simulink model "IDMF_datagenerator"  (R2022a)
settings: Solver=VariableStepAuto  StartTime=0.0  StopTime=30  FixedStep=0.05  RelTol=1e-3
PostLoadFcn:
  | %Add subfolders to path
  | addpath('virtualworld');
InitFcn:
  | startScript;
values from neighbouring files (symbols this model uses):
  angularVelocity = [0 0 -0.01]    [startScript.m]
  angularVelocityforLanding = [0 0 0]    [startScript.m]
  dronestartlocation = [-1.5 0 4]    [startScript.m]
  Dstar = -0.5    [startScript.m]
  finalHoverHeight = 2.5    [startScript.m]
  helipadLocation = [14 0.6 5]    [startScript.m]
  linearVelocity = [5 0.05 1]    [startScript.m]
  linearVelocityforHover = [0.65 0.05 0.3]    [startScript.m]
  windAVelocity = [0 0.1 0.1]    [startScript.m]
  windLVelocity = [0.1 0 0.3]    [startScript.m]
undefined symbols (not defined in the file or in its folder): fspecial, gcbh, Kanade, Lucas, Rec, SDTV, vrmfunc
libraries: visiontextngfix x11, visionconversions x9, visionanalysis x8, vrlib x7, slpidlib x3, sharedtransform x2, simulink x1
(part 2 of 3)

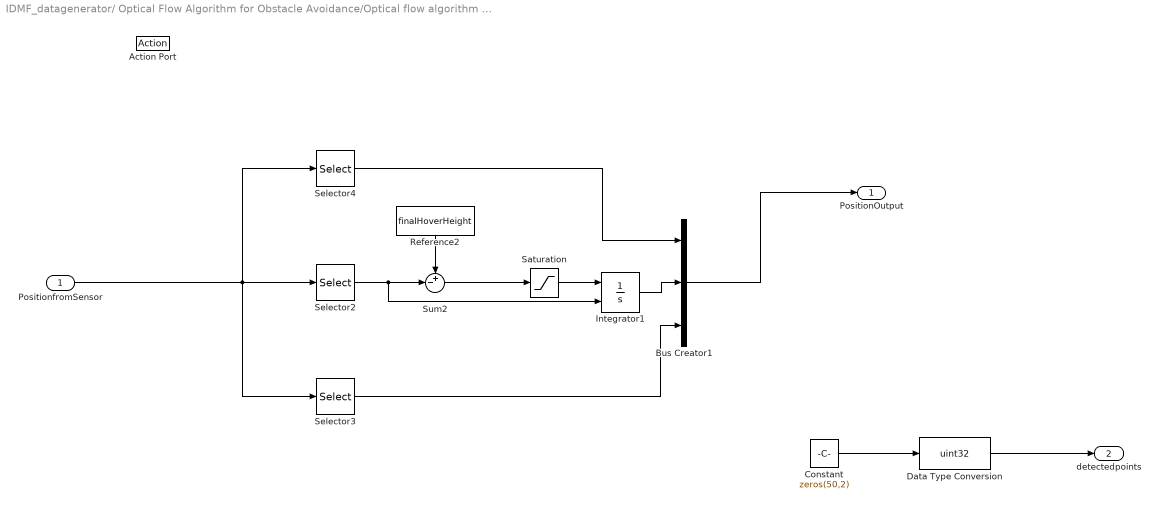
== system IDMF_datagenerator/ Optical Flow Algorithm for Obstacle Avoidance/Optical flow algorithm and PID Controller for landing/DronePositionEstimation.DroneLanding2 ==
  PositionfromSensor : Inport
  Action Port : ActionPort
      settings: CopyFcn=Stateflow.SLINSF.SimulinkMan.removeBlockPreDeleteFcn  PreDeleteFcn=Stateflow.SLINSF.SimulinkMan.unsafePredeleteFcn
  Bus Creator1 : BusCreator  Inputs=3
  Constant : Constant  Value=zeros(50,2)
  Data Type Conversion : DataTypeConversion  OutDataTypeStr=uint32  SaturateOnIntegerOverflow=off  RndMeth=Floor
  Integrator1 : Integrator  InitialConditionSource=external  LimitOutput=on  UpperSaturationLimit=5  LowerSaturationLimit=-5  ZeroCross=off
  Reference2 : Constant  Value=finalHoverHeight
  Saturation : Saturate  UpperLimit=5  LowerLimit=-5
  Selector2 : Selector  InputPortWidth=3  IndexOptions=Index vector (dialog)  Indices=[2]  OutputSizes=1
  Selector3 : Selector  InputPortWidth=3  IndexOptions=Index vector (dialog)  Indices=[3]  OutputSizes=1
  Selector4 : Selector  InputPortWidth=3  IndexOptions=Index vector (dialog)  Indices=[1]  OutputSizes=1
  Sum2 : Sum  Inputs=+-|
  PositionOutput : Outport
  detectedpoints : Outport  Port=2
      settings: VarSizeSig=Yes
  wires:
  Integrator1/1 -> Bus Creator1/2
  Saturation/1 -> Integrator1/1
  Bus Creator1/1 -> PositionOutput/1
  Selector2/1 -> Integrator1/2, Sum2/2
  Selector3/1 -> Bus Creator1/3
  PositionfromSensor/1 -> Selector3/1, Selector4/1, Selector2/1
  Reference2/1 -> Sum2/1
  Selector4/1 -> Bus Creator1/1
  Sum2/1 -> Saturation/1
  Constant/1 -> Data Type Conversion/1
  Data Type Conversion/1 -> detectedpoints/1

== system IDMF_datagenerator/ Optical Flow Algorithm for Obstacle Avoidance/Optical flow algorithm and PID Controller for landing/DronePositionEstimation.DroneLandingnoZ ==
  PositionfromSensor : Inport
  D_est : Inport  Port=2
  camera_d : Inport  Port=3
  linearVelocity : Inport  Port=4
  Action Port : ActionPort
      settings: CopyFcn=Stateflow.SLINSF.SimulinkMan.removeBlockPreDeleteFcn  PreDeleteFcn=Stateflow.SLINSF.SimulinkMan.unsafePredeleteFcn
  Landing : Subsystem
  Subsystem : Subsystem
  PositionOutput : Outport
  detectedpoints : Outport  Port=2  OutDataTypeStr=uint32
  wires:
  PositionfromSensor/1 -> Landing/1(In1)
  D_est/1 -> Landing/2(D_est)
  Landing/1(PositionOutput) -> PositionOutput/1
  camera_d/1 -> Subsystem/1(Input)
  Subsystem/1(Output) -> detectedpoints/1
  linearVelocity/1 -> Landing/3(linearVelocity)

== system IDMF_datagenerator/ Optical Flow Algorithm for Obstacle Avoidance/Optical flow algorithm and PID Controller for landing/DronePositionEstimation.OpticalFlowAlgorithm_ ==
  note: If the output from the Sign block is Positive, drone should move towards the left side, i.e. V_y is Negative. Also, if the output from the Sign block is Negative, drone will move towwars the right side..ie, V_y is Positive.
  note: Steering Linear Velocities
  OpticalFlowDiff : Inport
  Action Port : ActionPort
      settings: CopyFcn=Stateflow.SLINSF.SimulinkMan.removeBlockPreDeleteFcn  PreDeleteFcn=Stateflow.SLINSF.SimulinkMan.unsafePredeleteFcn
  Constant : Constant  Value=uint32(zeros(50,2))
  Constant1 : Constant  Value=linearVelocity
  Gain : Gain  Gain=[1 1 -1]
  Integrator2 : Integrator  InitialCondition=dronestartlocation
  Sign : Signum
  Switch1 : Switch  Criteria=u2 > Threshold  SaturateOnIntegerOverflow=off  InputSameDT=off
  PositionOutput : Outport
  detectedpoints : Outport  Port=2
      settings: VarSizeSig=Yes
  wires:
  OpticalFlowDiff/1 -> Sign/1
  Constant1/1 -> Switch1/3, Gain/1  "[V_X V_Z V_Y]"
  Switch1/1 -> Integrator2/1
  Gain/1 -> Switch1/1  "[V_X V_Z -1*V_Y]"
  Constant/1 -> detectedpoints/1
  Sign/1 -> Switch1/2
  Integrator2/1 -> PositionOutput/1

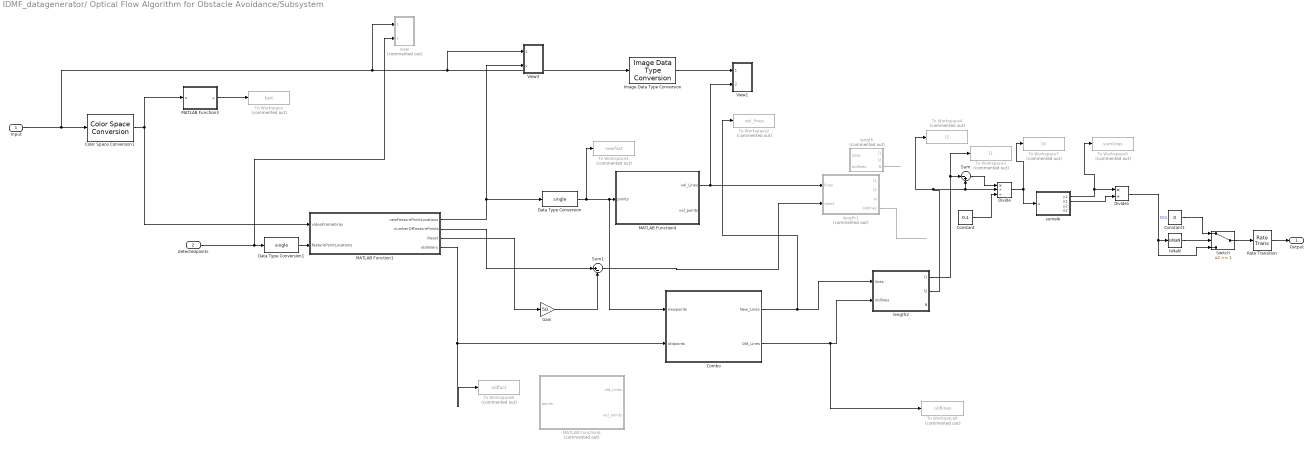
== system IDMF_datagenerator/ Optical Flow Algorithm for Obstacle Avoidance/Subsystem ==
  Input : Inport
  detectedpoints : Inport  Port=2
  Color Space Conversion1 : visionconversions/Color Space  Conversion  conversion=Obsolete  conversionActive=R'G'B' to intensity  wp_str=D65  rec=Rec. 601 (SDTV)  sys=1125/60/2:1  imagePorts=One multidimensional signal
  Combo : MATLAB Function  TreatAsAtomicUnit=on
  Constant : Constant  Value=0.1
  Constant1 : Constant  Value=0
  Data Type Conversion : DataTypeConversion  OutDataTypeStr=single  SaturateOnIntegerOverflow=off  RndMeth=Floor
  Data Type Conversion1 : DataTypeConversion  OutDataTypeStr=single  SaturateOnIntegerOverflow=off  RndMeth=Floor
  Divide : Product  Inputs=*//
  Divide1 : Product  Inputs=*/
  Gain : Gain  Gain=50
  Image Data Type Conversion : visionconversions/Image Data Type Conversion  outDT=single  isSigned=on  wordLen=16  numFracBits=0
      settings: SourceProductBaseCode=VP
  IsNaN : RelationalOperator  Operator=isNaN  OutDataTypeStr=boolean  RndMeth=Simplest  InputSameDT=off
  MATLAB Function1 : MATLAB Function  TreatAsAtomicUnit=on
  MATLAB Function3 : MATLAB Function  TreatAsAtomicUnit=on
  MATLAB Function4 : MATLAB Function  TreatAsAtomicUnit=on
  MATLAB Function6 : MATLAB Function  Commented=on  TreatAsAtomicUnit=on
  Rate Transition : RateTransition  OutPortSampleTime=0.1
  Sum : Sum  Inputs=|-+
  Sum1 : Sum  Inputs=|+-
  Switch : Switch  Threshold=1  SaturateOnIntegerOverflow=off  InputSameDT=off
  To Workspace : ToWorkspace  Commented=on  VariableName=fast  SaveFormat=Timeseries  SampleTime=-1
  To Workspace1 : ToWorkspace  Commented=on  VariableName=newfast  SaveFormat=Timeseries  SampleTime=-1
  To Workspace2 : ToWorkspace  Commented=on  VariableName=vel_lines  SaveFormat=Timeseries  SampleTime=-1
  To Workspace3 : ToWorkspace  Commented=on  VariableName=l1  SaveFormat=Timeseries  SampleTime=-1
  To Workspace4 : ToWorkspace  Commented=on  VariableName=l2  SaveFormat=Timeseries  SampleTime=-1
  To Workspace5 : ToWorkspace  Commented=on  VariableName=sumlines  SaveFormat=Timeseries  SampleTime=-1
  To Workspace6 : ToWorkspace  Commented=on  VariableName=oldlines  SaveFormat=Timeseries  SampleTime=-1
  To Workspace7 : ToWorkspace  Commented=on  VariableName=Di  SaveFormat=Timeseries  SampleTime=-1
  To Workspace8 : ToWorkspace  Commented=on  VariableName=oldfast  SaveFormat=Timeseries  SampleTime=-1
  View : Subsystem  Commented=on
  View1 : Subsystem
  View3 : Subsystem
  length : MATLAB Function  Commented=on  TreatAsAtomicUnit=on
  length1 : MATLAB Function  Commented=on  TreatAsAtomicUnit=on
  length2 : MATLAB Function  TreatAsAtomicUnit=on
  sumele : MATLAB Function  TreatAsAtomicUnit=on
  Output : Outport
  wires:
  Input/1 -> View/1(d_camera), View3/1(d_camera), Image Data Type Conversion/1, Color Space Conversion1/1
  Data Type Conversion/1 -> To Workspace1/1, Combo/1(newpoints), MATLAB Function4/1(points)
  MATLAB Function3/1(y) -> To Workspace/1
  detectedpoints/1 -> View/2(y), Data Type Conversion1/1
  Data Type Conversion1/1 -> MATLAB Function1/2(featurePointLocations)
  Color Space Conversion1/1 -> MATLAB Function1/1(videoFrameGray), MATLAB Function3/1(u)
  Image Data Type Conversion/1 -> View1/1(camera_d)
  Sum/1 -> Divide/1
  Constant/1 -> Divide/3
  Divide/1 -> sumele/1(u), To Workspace7/1
  Divide1/1 -> Switch/3, IsNaN/1  "Dca"
  sumele/1(y1) -> To Workspace5/1, Divide1/1
  sumele/2(n1) -> Divide1/2
  length/3(N) -> ?
  MATLAB Function1/2(numberOfFeaturePoints) -> Sum1/1
  MATLAB Function1/3(Reset) -> Gain/1
  Gain/1 -> Sum1/2
  Sum1/1 -> length1/2(reset)
  MATLAB Function4/1(vel_Lines) -> View1/2(vel_Lines), length1/1(lines)
  length1/4(oldlines) -> ?
  MATLAB Function1/4(oldInliers) -> To Workspace8/1, Combo/2(oldpoints)
  length2/1(l1) -> To Workspace3/1, Sum/1
  length2/2(l2) -> Divide/2, Sum/2, To Workspace4/1
  Combo/2(Old_Lines) -> To Workspace6/1, length2/2(oldlines)
  Combo/1(New_Lines) -> To Workspace2/1, length2/1(lines)
  MATLAB Function1/1(newFeaturePointLocations) -> View3/2(y), Data Type Conversion/1
  IsNaN/1 -> Switch/2
  Switch/1 -> Rate Transition/1
  Constant1/1 -> Switch/1
  Rate Transition/1 -> Output/1

== system IDMF_datagenerator/ Optical Flow Algorithm for Obstacle Avoidance/flowdiff ==
  image : Inport
  Delay1 : Delay
  FlowDifferences : MATLAB Function  TreatAsAtomicUnit=on
  Gain : Gain  Gain=1/10^3
  Sum1 : Sum  Inputs=+-
  Out1 : Outport
  Out2 : Outport  Port=2
  vleftflow : Outport  Port=3
  vrightflow : Outport  Port=4
  cmd : Outport  Port=5
  wires:
  Gain/1 -> Out2/1, Delay1/1, Sum1/1
  FlowDifferences/1(flowDifference) -> Gain/1
  Sum1/1 -> Out1/1
  FlowDifferences/3(vrightflow) -> vrightflow/1
  FlowDifferences/4(cmd) -> cmd/1
  Delay1/1 -> Sum1/2
  image/1 -> FlowDifferences/1(image)
  FlowDifferences/2(vleftflow) -> vleftflow/1

== system IDMF_datagenerator/ Optical Flow Algorithm for Obstacle Avoidance/flowdiff_down ==
  image : Inport
  Delay : Delay  DelayLength=1
  Delay2 : Delay  DelayLength=1
  FlowDifferences1 : MATLAB Function  TreatAsAtomicUnit=on
  FlowDifferences2 : MATLAB Function  TreatAsAtomicUnit=on
  Gain1 : Gain  Gain=1/10^3
  Gain2 : Gain  Gain=1/10^3
  Sum : Sum  Inputs=+-
  Sum2 : Sum  Inputs=+-
  ofd_up_d : Outport
  flowdiff_down : Outport  Port=2
  ofd_d : Outport  Port=3
  flowup_down : Outport  Port=4
  wires:
  image/1 -> FlowDifferences2/1(image), FlowDifferences1/1(image)
  Gain1/1 -> flowdiff_down/1, Sum/1, Delay/1  "flowdiff_down"
  Gain2/1 -> flowup_down/1, Delay2/1, Sum2/1  "flowup_down"
  FlowDifferences1/1(flowDifference) -> Gain1/1  "flowdiff_down"
  Delay/1 -> Sum/2
  FlowDifferences2/1(flowDifference) -> Gain2/1  "flowup_down"
  Sum2/1 -> ofd_up_d/1  "ofd_up_d"
  Delay2/1 -> Sum2/2
  Sum/1 -> ofd_d/1  "ofd_d"

== system IDMF_datagenerator/Optical Flow Lines Calculation/Optical Flow Lines ==
  vel.Values : Inport
  Optical Flow Lines : MATLAB Function  TreatAsAtomicUnit=on
  vel.Lines : Outport
  wires:
  Optical Flow Lines/1(vel_Lines) -> vel.Lines/1
  vel.Values/1 -> Optical Flow Lines/1(vel_Values)

== system IDMF_datagenerator/Optical Flow Lines Calculation/Optical Flow Lines1 ==
  vel.Values : Inport
  Optical Flow Lines : MATLAB Function  TreatAsAtomicUnit=on
  vel.Lines : Outport
  wires:
  Optical Flow Lines/1(vel_Lines) -> vel.Lines/1
  vel.Values/1 -> Optical Flow Lines/1(vel_Values)

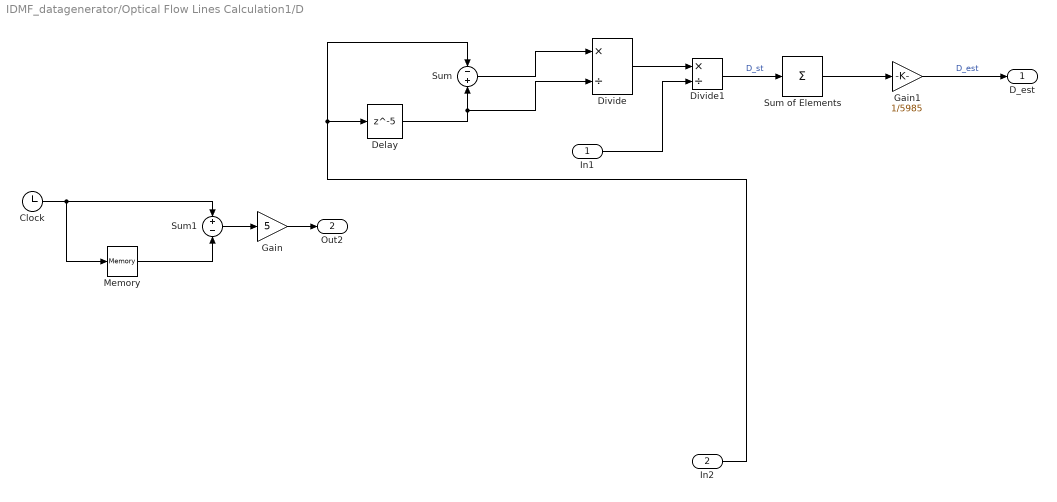
== system IDMF_datagenerator/Optical Flow Lines Calculation1/D ==
  In1 : Inport
  In2 : Inport  Port=2
  Clock : Clock
  Delay : Delay  DelayLength=5
  Divide : Product  Inputs=*/
  Divide1 : Product  Inputs=*/
  Gain : Gain  Gain=5
  Gain1 : Gain  Gain=1/5985
  Memory : Memory
  Sum : Sum  Inputs=-+
  Sum of Elements : Sum  Inputs=+
  Sum1 : Sum  Inputs=+-
  D_est : Outport
  Out2 : Outport  Port=2
  wires:
  Divide/1 -> Divide1/1
  Clock/1 -> Memory/1, Sum1/1
  Sum1/1 -> Gain/1
  Delay/1 -> Divide/2, Sum/2
  Sum/1 -> Divide/1
  Sum of Elements/1 -> Gain1/1
  In2/1 -> Delay/1, Sum/1
  Memory/1 -> Sum1/2
  Divide1/1 -> Sum of Elements/1  "D_st"
  In1/1 -> Divide1/2
  Gain/1 -> Out2/1
  Gain1/1 -> D_est/1  "D_est"

== system IDMF_datagenerator/Optical Flow Lines Calculation1/View ==
  d_camera : Inport
  In2 : Inport  Port=2
  Data Type Conversion : DataTypeConversion  OutDataTypeStr=int32  SaturateOnIntegerOverflow=off  RndMeth=Floor
  Draw Markers1 : visiontextngfix/Draw Markers  shape=X-mark  size=3  fill=off  fillClrSource=Specify via dialog  display=User-specified value  intensity=200  color=[255 0 0]  opacity=0.6  viewport=Entire image  antialiasing=off  inType=Obsolete  imagePorts=One multidimensional signal  roundingMode=Floor  overflowMode=off  memoryMode=Specify word length  memoryWordLength=16  memoryFracLength=15  prodOutputMode=Binary point scaling  prodOutputWordLength=32  prodOutputFracLength=14
      settings: SourceProductBaseCode=VP
  points for ownline : VideoViewer  FigPos=[132 616 560 453]
  wires:
  In2/1 -> Data Type Conversion/1
  Draw Markers1/1 -> points for ownline/1
  d_camera/1 -> Draw Markers1/1
  Data Type Conversion/1 -> Draw Markers1/2

== system IDMF_datagenerator/Optical Flow Lines Calculation1/View1 ==
  In1 : Inport
  In2 : Inport  Port=2
  Data Type Conversion : DataTypeConversion  OutDataTypeStr=int32  SaturateOnIntegerOverflow=off  RndMeth=Floor
  Draw Shapes2 : visiontextngfix/Draw Shapes  shape=Lines  fill=off  lineWidth=1  fillClrSource=Specify via dialog  display=User-specified value  intensity=200  color=[255 255 0]  opacity=0.6  viewport=Entire image  antialiasing=off  inType=Obsolete  imagePorts=One multidimensional signal  roundingMode=Floor  overflowMode=off  memoryMode=Specify word length  memoryWordLength=16  prodOutputMode=Binary point scaling  prodOutputWordLength=32  prodOutputFracLength=14  memoryFracLength=15
  owncode lines : VideoViewer  FigPos=[594 703 418 304]
  wires:
  Draw Shapes2/1 -> owncode lines/1
  In1/1 -> Draw Shapes2/1
  Data Type Conversion/1 -> Draw Shapes2/2
  In2/1 -> Data Type Conversion/1

== system IDMF_datagenerator/ Optical Flow Algorithm for Obstacle Avoidance/Optical flow algorithm and PID Controller for landing/DronePositionEstimation.DroneLandingnoZ/Landing ==
  note: Steering Linear Velocities
  In1 : Inport
  D_est : Inport  Port=2
  linearVelocity : Inport  Port=3
  Bus Creator1 : BusCreator  Inputs=3
  Constant : Constant  Value=linearVelocity
  Integrator2 : Integrator  InitialConditionSource=external  InitialCondition=dronestartlocation
  Manual Switch : ManualSwitch  CurrentSetting=0
  Manual Switch1 : ManualSwitch  CurrentSetting=0
  Selector2 : Selector  InputPortWidth=3  IndexOptions=Index vector (dialog)  Indices=[2]  OutputSizes=1
  Selector3 : Selector  InputPortWidth=3  IndexOptions=Index vector (dialog)  Indices=[3]  OutputSizes=1
  Selector4 : Selector  InputPortWidth=3  IndexOptions=Index vector (dialog)  Indices=[1]  OutputSizes=1
  Subsystem : Subsystem
  PositionOutput : Outport
  wires:
  D_est/1 -> Subsystem/2(D_est)
  Selector4/1 -> Bus Creator1/1
  Selector3/1 -> Bus Creator1/3
  Subsystem/1(Z) -> Bus Creator1/2
  Bus Creator1/1 -> PositionOutput/1
  Selector2/1 -> Subsystem/1(InitialZ)
  Manual Switch/1 -> Integrator2/1  "[V_X V_Z -1*V_Y]"
  Constant/1 -> Manual Switch/1
  Integrator2/1 -> Manual Switch1/1
  linearVelocity/1 -> Manual Switch/2
  Manual Switch1/1 -> Selector4/1, Selector3/1, Selector2/1
  In1/1 -> Integrator2/2, Manual Switch1/2

== system IDMF_datagenerator/ Optical Flow Algorithm for Obstacle Avoidance/Optical flow algorithm and PID Controller for landing/DronePositionEstimation.DroneLandingnoZ/Subsystem ==
  Input : Inport
  Color Space Conversion1 : visionconversions/Color Space  Conversion  conversion=Obsolete  conversionActive=R'G'B' to intensity  wp_str=D65  rec=Rec. 601 (SDTV)  sys=1125/60/2:1  imagePorts=One multidimensional signal
  Corner Detection : visionanalysis/Corner Detection  method=Local intensity comparison (Rosen & Drummond)  factor=0.04  filter=fspecial('gaussian', [1 5], 1.5)  thrInten=0.1  thrAngle=157.5  output=Obsolete9b  outputInUse=Corner location  maxNum=50  thrMetric=0.005  neighborSize=[15 15]  isOutVarDim=off  roundingMode=Floor  overflowMode=off  firstCoeffMode=Specify word length  firstCoeffWordLength=16  firstCoeffFracLength=16  prodOutputMode=Binary point scaling  prodOutputWordLength=32  prodOutputFracLength=0  accumMode=Binary point scaling  accumWordLength=32  accumFracLength=0  memoryMode=Binary point scaling  memoryWordLength=32  memoryFracLength=0
      settings: SourceProductBaseCode=VP
  Corner Detection1 : visionanalysis/Corner Detection  method=Local intensity comparison (Rosen & Drummond)  factor=0.04  filter=fspecial('gaussian', [1 5], 1.5)  thrInten=0.1  thrAngle=112.5  output=Obsolete9b  outputInUse=Corner location  maxNum=50  thrMetric=0.0005  neighborSize=[25 25]  isOutVarDim=off  roundingMode=Floor  overflowMode=off  firstCoeffMode=Specify word length  firstCoeffWordLength=16  firstCoeffFracLength=16  prodOutputMode=Binary point scaling  prodOutputWordLength=32  prodOutputFracLength=0  accumMode=Binary point scaling  accumWordLength=32  accumFracLength=0  memoryMode=Binary point scaling  memoryWordLength=32  memoryFracLength=0
      settings: SourceProductBaseCode=VP
  Output : Outport
  wires:
  Input/1 -> Color Space Conversion1/1
  Color Space Conversion1/1 -> Corner Detection/1
  Corner Detection/1 -> Output/1

== system IDMF_datagenerator/ Optical Flow Algorithm for Obstacle Avoidance/Subsystem/View ==
  d_camera : Inport
  y : Inport  Port=2
  Data Type Conversion : DataTypeConversion  OutDataTypeStr=int32  SaturateOnIntegerOverflow=off  RndMeth=Floor
  Draw Markers1 : visiontextngfix/Draw Markers  shape=X-mark  size=3  fill=off  fillClrSource=Specify via dialog  display=User-specified value  intensity=200  color=[255 0 0]  opacity=0.6  viewport=Entire image  antialiasing=off  inType=Obsolete  imagePorts=One multidimensional signal  roundingMode=Floor  overflowMode=off  memoryMode=Specify word length  memoryWordLength=16  memoryFracLength=15  prodOutputMode=Binary point scaling  prodOutputWordLength=32  prodOutputFracLength=14
      settings: SourceProductBaseCode=VP
  points from new : VideoViewer  FigPos=[1 1038 1920 938]
  wires:
  y/1 -> Data Type Conversion/1
  Draw Markers1/1 -> points from new/1
  d_camera/1 -> Draw Markers1/1
  Data Type Conversion/1 -> Draw Markers1/2

== system IDMF_datagenerator/ Optical Flow Algorithm for Obstacle Avoidance/Subsystem/View1 ==
  camera_d : Inport
  vel_Lines : Inport  Port=2
  Detected lines : VideoViewer  FigPos=[1 1078 1184 528]
  Draw Shapes2 : visiontextngfix/Draw Shapes  shape=Lines  fill=off  lineWidth=1  fillClrSource=Specify via dialog  display=User-specified value  intensity=200  color=[255 255 0]  opacity=0.6  viewport=Entire image  antialiasing=off  inType=Obsolete  imagePorts=One multidimensional signal  roundingMode=Floor  overflowMode=off  memoryMode=Specify word length  memoryWordLength=16  prodOutputMode=Binary point scaling  prodOutputWordLength=32  prodOutputFracLength=14  memoryFracLength=15
  wires:
  camera_d/1 -> Draw Shapes2/1
  vel_Lines/1 -> Draw Shapes2/2
  Draw Shapes2/1 -> Detected lines/1

== system IDMF_datagenerator/ Optical Flow Algorithm for Obstacle Avoidance/Subsystem/View3 ==
  d_camera : Inport
  y : Inport  Port=2
  Data Type Conversion : DataTypeConversion  OutDataTypeStr=int32  SaturateOnIntegerOverflow=off  RndMeth=Floor
  Draw Markers1 : visiontextngfix/Draw Markers  shape=X-mark  size=3  fill=off  fillClrSource=Specify via dialog  display=User-specified value  intensity=200  color=[255 0 0]  opacity=0.6  viewport=Entire image  antialiasing=off  inType=Obsolete  imagePorts=One multidimensional signal  roundingMode=Floor  overflowMode=off  memoryMode=Specify word length  memoryWordLength=16  memoryFracLength=15  prodOutputMode=Binary point scaling  prodOutputWordLength=32  prodOutputFracLength=14
      settings: SourceProductBaseCode=VP
  points from new : VideoViewer  FigPos=[1172 788 606 520]
  wires:
  y/1 -> Data Type Conversion/1
  Draw Markers1/1 -> points from new/1
  d_camera/1 -> Draw Markers1/1
  Data Type Conversion/1 -> Draw Markers1/2

== system IDMF_datagenerator/ Optical Flow Algorithm for Obstacle Avoidance/Optical flow algorithm and PID Controller for landing/DronePositionEstimation.DroneLandingnoZ/Landing/Subsystem ==
  InitialZ : Inport
  D_est : Inport  Port=2
  Subsystem : Subsystem
  Subsystem1 : Subsystem
  Z : Outport
  wires:
  InitialZ/1 -> Subsystem/1(InitialZ), Subsystem1/1(InitialZ)
  D_est/1 -> Subsystem/2(D_est)
  Subsystem/1(Z) -> Subsystem1/2(calcZ)
  Subsystem/2(resetp) -> Subsystem1/3(resetp)
  Subsystem1/1(Z) -> Z/1

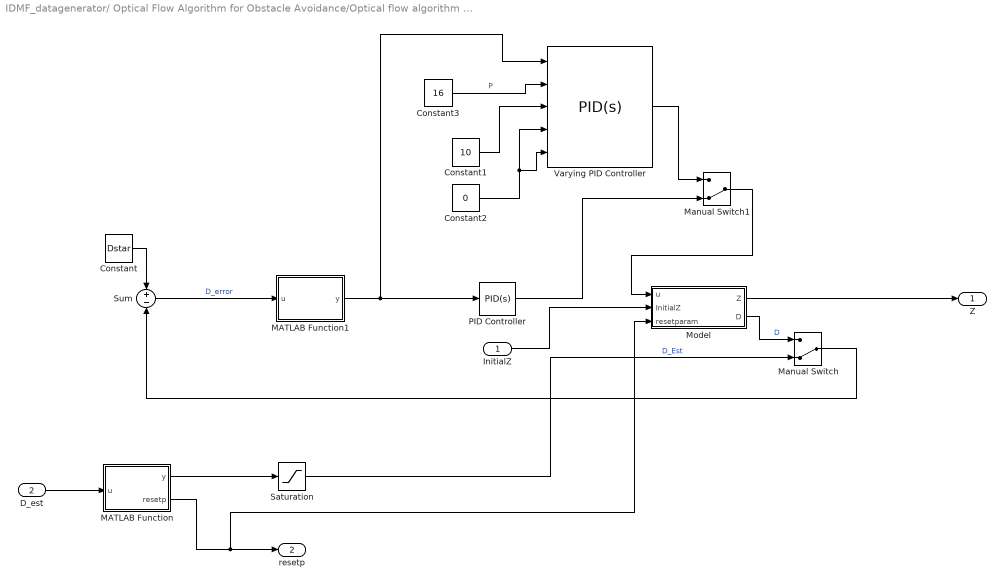
== system IDMF_datagenerator/ Optical Flow Algorithm for Obstacle Avoidance/Optical flow algorithm and PID Controller for landing/DronePositionEstimation.DroneLandingnoZ/Landing/Subsystem/Subsystem ==
  InitialZ : Inport
  D_est : Inport  Port=2
  Constant : Constant  Value=Dstar
  Constant1 : Constant  Value=10
  Constant2 : Constant  Value=0
  Constant3 : Constant  Value=16
  MATLAB Function : MATLAB Function  TreatAsAtomicUnit=on
  MATLAB Function1 : MATLAB Function  TreatAsAtomicUnit=on
  Manual Switch : ManualSwitch  CurrentSetting=0
  Manual Switch1 : ManualSwitch  CurrentSetting=0
  Model : Subsystem
  PID Controller : slpidlib/PID Controller  Controller=PID  Form=Parallel  TimeDomain=Continuous-time  UseExternalTs=off  SampleTime=-1  IntegratorMethod=Forward Euler  FilterMethod=Forward Euler  ControllerParametersSource=internal  P=16  I=10  UseKiTs=off  D=0  N=100  UseFilter=on  TunerSelectOption=Transfer Function Based (PID Tuner App)  InitialConditionSource=internal  InitialConditionForIntegrator=0  InitialConditionForFilter=0  DifferentiatorICPrevScaledInput=0  ExternalReset=none  TrackingMode=off  Kt=1  LimitOutput=off  SatLimitsSource=internal  UpperSaturationLimit=inf  LowerSaturationLimit=-inf  LinearizeAsGain=on  AntiWindupMode=none  Kb=1  POutMin=[]  POutMax=[]  IOutMin=[]  IOutMax=[]  DOutMin=[]  DOutMax=[]  NOutMin=[]  NOutMax=[]  SumOutMin=[]  SumOutMax=[]  SaturationOutMin=[]  SaturationOutMax=[]  PParamMin=[]  PParamMax=[]  IParamMin=[]  IParamMax=[]  DParamMin=[]  DParamMax=[]  NParamMin=[]  NParamMax=[]  KbParamMin=[]  KbParamMax=[]  KtParamMin=[]  KtParamMax=[]  KbOutMin=[]  KbOutMax=[]  KtOutMin=[]  KtOutMax=[]  IntegratorOutMin=[]  IntegratorOutMax=[]  FilterOutMin=[]  FilterOutMax=[]  SumI1OutMin=[]  SumI1OutMax=[]  SumI2OutMin=[]  SumI2OutMax=[]  SumI3OutMin=[]  SumI3OutMax=[]  SumI4OutMin=[]  SumI4OutMax=[]  SumDOutMin=[]  SumDOutMax=[]  DifferentiatorOutMin=[]  DifferentiatorOutMax=[]  FilterDiffOutCoefMin=[]  FilterDiffOutCoefMax=[]  ReciprocalOutMin=[]  ReciprocalOutMax=[]  SumDenOutMin=[]  SumDenOutMax=[]  SumNumOutMin=[]  SumNumOutMax=[]  DivideOutMin=[]  DivideOutMax=[]  UdiffTsProdOutMin=[]  UdiffTsProdOutMax=[]  NTsProdOutMin=[]  NTsProdOutMax=[]  UintegralTsProdOutMin=[]  UintegralTsProdOutMax=[]  UngainTsProdOutMin=[]  UngainTsProdOutMax=[]  IntegratorContinuousStateAttributes=''  IntegratorStateMustResolveToSignalObject=off  IntegratorRTWStateStorageClass=Auto  FilterContinuousStateAttributes=''  FilterStateMustResolveToSignalObject=off  FilterRTWStateStorageClass=Auto  ParallelPVariant=InternalParameters  IdealPVariant=Disabled  IVariant=InternalParameters  DVariant=InternalParameters  IntegratorVariant=Continuous  SatVariant=Disabled  AWVariant=Passthrough  PCopyVariant=Disabled  TRVariant=Disabled  FdbkBlocksVariant=Forward  IdealPFdbkVariant=Disabled  SatFdbkVariant=Disabled  DerivativeFilterVariant=ContFilter  NVariant=InternalParameters  NCopyVariant=Disabled  FilterICVariant=InternalICsFilter  IntegratorICVariant=InternalICs  ExternalResetVariant=Disabled  TRSumVariant=Passthrough  SumFdbkVariant=Disabled  SumVariant=Sum_PID  TsampFilterVariant=InternalTs  TsampNgainVariant=Passthrough  TsampIntegralVariant=Passthrough  ExternalSaturationOutDataTypeStr=Inherit: Same as second input  aMode=0
  Saturation : Saturate  UpperLimit=1  LowerLimit=-1
  Sum : Sum  Inputs=+-
  Varying PID Controller : slpidlib/PID Controller  Controller=PID  Form=Parallel  TimeDomain=Continuous-time  UseExternalTs=off  SampleTime=-1  IntegratorMethod=Forward Euler  FilterMethod=Forward Euler  ControllerParametersSource=external  P=1  I=1  UseKiTs=off  D=0  N=100  UseFilter=on  TunerSelectOption=Transfer Function Based (PID Tuner App)  InitialConditionSource=internal  InitialConditionForIntegrator=0  InitialConditionForFilter=0  DifferentiatorICPrevScaledInput=0  ExternalReset=none  TrackingMode=off  Kt=1  LimitOutput=off  SatLimitsSource=internal  UpperSaturationLimit=inf  LowerSaturationLimit=-inf  LinearizeAsGain=on  AntiWindupMode=none  Kb=1  POutMin=[]  POutMax=[]  IOutMin=[]  IOutMax=[]  DOutMin=[]  DOutMax=[]  NOutMin=[]  NOutMax=[]  SumOutMin=[]  SumOutMax=[]  SaturationOutMin=[]  SaturationOutMax=[]  PParamMin=[]  PParamMax=[]  IParamMin=[]  IParamMax=[]  DParamMin=[]  DParamMax=[]  NParamMin=[]  NParamMax=[]  KbParamMin=[]  KbParamMax=[]  KtParamMin=[]  KtParamMax=[]  KbOutMin=[]  KbOutMax=[]  KtOutMin=[]  KtOutMax=[]  IntegratorOutMin=[]  IntegratorOutMax=[]  FilterOutMin=[]  FilterOutMax=[]  SumI1OutMin=[]  SumI1OutMax=[]  SumI2OutMin=[]  SumI2OutMax=[]  SumI3OutMin=[]  SumI3OutMax=[]  SumI4OutMin=[]  SumI4OutMax=[]  SumDOutMin=[]  SumDOutMax=[]  DifferentiatorOutMin=[]  DifferentiatorOutMax=[]  FilterDiffOutCoefMin=[]  FilterDiffOutCoefMax=[]  ReciprocalOutMin=[]  ReciprocalOutMax=[]  SumDenOutMin=[]  SumDenOutMax=[]  SumNumOutMin=[]  SumNumOutMax=[]  DivideOutMin=[]  DivideOutMax=[]  UdiffTsProdOutMin=[]  UdiffTsProdOutMax=[]  NTsProdOutMin=[]  NTsProdOutMax=[]  UintegralTsProdOutMin=[]  UintegralTsProdOutMax=[]  UngainTsProdOutMin=[]  UngainTsProdOutMax=[]  IntegratorContinuousStateAttributes=''  IntegratorStateMustResolveToSignalObject=off  IntegratorRTWStateStorageClass=Auto  FilterContinuousStateAttributes=''  FilterStateMustResolveToSignalObject=off  FilterRTWStateStorageClass=Auto  ParallelPVariant=ExternalParameters  IdealPVariant=Disabled  IVariant=ExternalParameters  DVariant=ExternalParameters  IntegratorVariant=Continuous  SatVariant=Disabled  AWVariant=Passthrough  PCopyVariant=Disabled  TRVariant=Disabled  FdbkBlocksVariant=Forward  IdealPFdbkVariant=Disabled  SatFdbkVariant=Disabled  DerivativeFilterVariant=ContFilter  NVariant=ExternalParameters  NCopyVariant=Disabled  FilterICVariant=InternalICsFilter  IntegratorICVariant=InternalICs  ExternalResetVariant=Disabled  TRSumVariant=Passthrough  SumFdbkVariant=Disabled  SumVariant=Sum_PID  TsampFilterVariant=InternalTs  TsampNgainVariant=Passthrough  TsampIntegralVariant=Passthrough  ExternalSaturationOutDataTypeStr=Inherit: Same as second input  aMode=0
  Z : Outport
  resetp : Outport  Port=2
  wires:
  Sum/1 -> MATLAB Function1/1(u)  "D_error"
  Model/2(D) -> Manual Switch/1  "D"
  Model/1(Z) -> Z/1
  MATLAB Function1/1(y) -> Varying PID Controller/1, PID Controller/1
  InitialZ/1 -> Model/2(InitialZ)
  PID Controller/1 -> Manual Switch1/2
  Constant/1 -> Sum/1
  Manual Switch/1 -> Sum/2
  D_est/1 -> MATLAB Function/1(u)
  MATLAB Function/1(y) -> Saturation/1
  Saturation/1 -> Manual Switch/2  "D_Est"
  MATLAB Function/2(resetp) -> Model/3(resetparam), resetp/1
  Constant1/1 -> Varying PID Controller/3
  Constant2/1 -> Varying PID Controller/5, Varying PID Controller/4
  Constant3/1 -> Varying PID Controller/2  "P"
  Varying PID Controller/1 -> Manual Switch1/1
  Manual Switch1/1 -> Model/1(u)

== system IDMF_datagenerator/ Optical Flow Algorithm for Obstacle Avoidance/Optical flow algorithm and PID Controller for landing/DronePositionEstimation.DroneLandingnoZ/Landing/Subsystem/Subsystem1 ==
  InitialZ : Inport
  calcZ : Inport  Port=2
  resetp : Inport  Port=3
  Compare To Constant : simulink/Logic and Bit Operations/Compare To Constant  relop=>  const=0  OutDataTypeStr=boolean
  First Order Hold : FirstOrderHold  InitialOutput=finalHoverHeight  ErrorTolerance=inf  AllowContinuousInput=on
  MATLAB Function : MATLAB Function  TreatAsAtomicUnit=on
  Stop Simulation : Stop
  Z : Outport
  wires:
  resetp/1 -> MATLAB Function/1(resetp)
  InitialZ/1 -> MATLAB Function/3(currentz)
  calcZ/1 -> MATLAB Function/2(calcz)
  MATLAB Function/2(stp) -> Compare To Constant/1
  Compare To Constant/1 -> Stop Simulation/1
  MATLAB Function/3(x1) -> ?
  MATLAB Function/1(opz) -> First Order Hold/1
  First Order Hold/1 -> Z/1

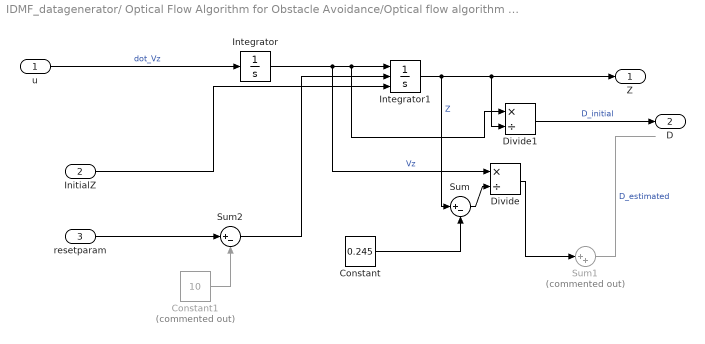
== system IDMF_datagenerator/ Optical Flow Algorithm for Obstacle Avoidance/Optical flow algorithm and PID Controller for landing/DronePositionEstimation.DroneLandingnoZ/Landing/Subsystem/Subsystem/Model ==
  u : Inport
  InitialZ : Inport  Port=2
  resetparam : Inport  Port=3
  Constant : Constant  Value=0.245
  Constant1 : Constant  Commented=on  Value=10
  Divide : Product  Inputs=*/
  Divide1 : Product  Inputs=*/
  Integrator : Integrator  InitialCondition=linearVelocityforHover(2)
  Integrator1 : Integrator  ExternalReset=falling  InitialConditionSource=external
  Sum : Sum  Inputs=|+-
  Sum1 : Sum  Commented=on  Inputs=|++
  Sum2 : Sum  Inputs=|+-
  Z : Outport
  D : Outport  Port=2
  wires:
  u/1 -> Integrator/1  "dot_Vz"
  Integrator/1 -> Divide/1, Divide1/1, Integrator1/1  "Vz"
  Integrator1/1 -> Sum/1, Divide1/2, Z/1  "Z"
  Divide/1 -> Sum1/1
  InitialZ/1 -> Integrator1/3
  Constant/1 -> Sum/2
  Sum/1 -> Divide/2
  Sum1/1 -> ?  "D_estimated"
  Divide1/1 -> D/1  "D_initial"
  Sum2/1 -> Integrator1/2
  resetparam/1 -> Sum2/1
  Constant1/1 -> Sum2/2

== matlab function IDMF_datagenerator/Optical Flow Lines Calculation1/Optical Flow Lines3 ==
  settings: updateMethod=DISCRETE
  data: vel_Values input; vel_Lines output; scaleFactor input size=1
function vel_Lines=OpticalFlowLines(vel_Values, scaleFactor) 

% Generates the coordinate points of optical flow lines

persistent first_time;
persistent X;
persistent Y;
persistent RV;
persistent CV;
if isempty(first_time)
    first_time     = 1;
    %% user may change the following three parameters
    borderOffset   = 5;
    decimFactorRow = 5;
    decimFactorCol = 5;    
    %%
    [R C] = size(vel_Values);
    RV = borderOffset:decimFactorRow:(R-borderOffset);   
    CV = borderOffset:decimFactorCol:(C-borderOffset);
    [Y X] = meshgrid(CV,RV);
end

tmp = vel_Values(RV,CV);
tmp = tmp.*scaleFactor;
vel_Lines = [Y(:), X(:), Y(:)+real(tmp(:)),  X(:)+imag(tmp(:))];

== matlab function IDMF_datagenerator/ Optical Flow Algorithm for Obstacle Avoidance/flowdiff_down/FlowDifferences1 ==
  data: flowDifference output; image input
function flowDifference = calculatethedifference(image)

% Image Preprocessing
image = flip(image, 1);

% Image Width
width = size(image,2);

% Calculate optical flow on right-half and the left-half of the image
VLeftFlow = image(:, 1:width/2); 
VRightFlow = image(:, width/2:width);

% Sum to get the total Optical Flow on the right-half and on left-half
vleftflow = sum(VLeftFlow(:));
vrightflow = sum(VRightFlow(:));

% Find the difference of the flow between the two halves
flowDifference = (vleftflow - vrightflow);

% Steer in the direction that has less optical flow which implies less 
% obstacles

== stateflow chart IDMF_datagenerator/ Optical Flow Algorithm for Obstacle Avoidance/Optical flow algorithm and PID Controller for landing ==
  settings: sampleTime=0.01
  state DronePositionEstimation [parallel]
    settings: executionOrder=1
    note: Controller for position is divided into three states:
        | Navigate left right based on optical flow lines
        | 2. Navigate the drone to hover over helipadLocation using PID controller
        | 3. Landing on the helipad from the height the drone was hovering at
    state DroneHover
    state OpticalFlowAlgorithm_
    state DroneLandingnoZ
    state DroneLanding2
    state DroneHover1
    (default) -> DronePositionEstimation.OpticalFlowAlgorithm_
    (junction 211) -> DroneHover
    DroneHover1 -> (junction 211) : [abs(xLocation-14) <= 0.25]
    DroneHover -> (junction 209) : [abs(PositionfromSensor(3)-5) <= 0.2...
        | && abs(xLocation-14) <= 0.26]
    (junction 209) -> DroneLandingnoZ
    DronePositionEstimation.OpticalFlowAlgorithm_ -> (junction 243) : [xLocation > 13]
    (junction 243) -> DroneLanding2
    DroneLanding2 -> DroneHover1 : [abs(zLocation-finalHoverHeight) <= 0.005]
  state ControlAlgorithm_ [parallel] [commented out]
  state DroneLanding [parallel] [commented out]
  state DroneLanding1 [parallel] [commented out]
  state DroneLanding_ [parallel] [commented out]
  state DroneLanding1 [parallel] [commented out]
  note: condition to switch to drone landing:
      |
      | [abs(yLocation-helipadLocation(3)) <= delta...
      | && abs(xLocation-helipadLocation(1)) <= delta]
      | [abs(zLocation-finalHoverHeight) <= 0.05]
      | ofd>470 for -1.5 0 0
      | [abs(ofd_d)>0.4]
      | [ofd<-1 && xLocation > switchingXLimit]
      | [ofd_d>2.2]
      | [abs(ofd_d)>2.5] for -1.5 0 0
      | [abs(ofd_d)>1.9] for -1.5 0 4
      | [abs(ofd_d)<=0.006 && abs(ofd_up_d)<=0.04]
      | [abs(ofd_d)<=0.01 && abs(ofd_up_d)<=0.6]
      |
      |
      | [abs(data)-abs(flowDifference)<=0.05]
  state DroneOrientationEstimation [parallel]
    settings: executionOrder=2
    note: Controller for orientation is divided into two parts:
        | Navigate left right based on optical flow lines
        | Constant angular velocity to move to helipadLocation
    state OpticalFlowAlgorithm_
    state ControlAlgorithm_
    (default) -> DroneOrientationEstimation.OpticalFlowAlgorithm_
    DroneOrientationEstimation.OpticalFlowAlgorithm_ -> (junction 133) : [xLocation > 13]
    (junction 133) -> DroneOrientationEstimation.ControlAlgorithm_ : after(0.01,sec)
  note: for clear helipad:
      | [abs(flowup_down)<=0.115 && abs(flowdiff_down)<=0.035]
      | after(1.25,sec)
      |
      | for concentric helipad:
      | [abs(flowup_down)<=0.33 && abs(flowdiff_down)<=0.22]
      | ofd<-1000 &&
      | [abs(ofd_d)>1.9]
  data: sf_internal_action_state_placeholder_data local double size=1 =0; sf_internal_action_state_placeholder_data local double size=1 =0; sf_internal_action_state_placeholder_data local double size=1 =0; sf_internal_action_state_placeholder_data local double size=1 =0; sf_internal_action_state_placeholder_data local double size=1 =0; sf_internal_action_state_placeholder_data local double size=1 =0; sf_internal_action_state_placeholder_data local double size=1 =0; sf_internal_action_state_placeholder_data local double size=1 =0; sf_internal_action_state_placeholder_data local double size=1 =0; sf_internal_action_state_placeholder_data local double size=1 =0; sf_internal_action_state_placeholder_data local double size=1 =0; sf_internal_action_state_placeholder_data local double size=1 =0; linearVelocity input; angularVelocity input; OpticalFlowDiff input; D_est input; ofd_up_d input; OrientationOutput output; zLocation input; PositionfromSensor input double; PositionOutput output; InitialCondition input; switchingXLimit local double; flowdiff_down input; finalHoverHeight input; xLocation input; camera_d input; ofd input; ofd_d input; flowup_down input; detectedpoints output size=[50 2]

== matlab function IDMF_datagenerator/Optical Flow Lines Calculation/Optical Flow Lines1/Optical Flow Lines ==
  data: vel_Values input; vel_Lines output; scaleFactor parameter size=1
function vel_Lines=OpticalFlowLines(vel_Values, scaleFactor) 

% Generates the coordinate points of optical flow lines

persistent first_time;
persistent X;
persistent Y;
persistent RV;
persistent CV;
if isempty(first_time)
    first_time     = 1;
    %% user may change the following three parameters
    borderOffset   = 5;
    decimFactorRow = 5;
    decimFactorCol = 5;    
    %%
    [R C] = size(vel_Values);
    RV = borderOffset:decimFactorRow:(R-borderOffset);   
    CV = borderOffset:decimFactorCol:(C-borderOffset);
    [Y X] = meshgrid(CV,RV);
end

tmp = vel_Values(RV,CV);
tmp = tmp.*scaleFactor;
vel_Lines = [Y(:), X(:), Y(:)+real(tmp(:)), X(:)+imag(tmp(:))];

== matlab function IDMF_datagenerator/Optical Flow Lines Calculation1/Optical Flow Lines2 ==
  settings: updateMethod=DISCRETE
  data: vel_Values input; vel_Lines output; scaleFactor input size=1
function vel_Lines=OpticalFlowLines(vel_Values, scaleFactor) 

% Generates the coordinate points of optical flow lines

persistent first_time;
persistent X;
persistent Y;
persistent RV;
persistent CV;
if isempty(first_time)
    first_time     = 1;
    %% user may change the following three parameters
    borderOffset   = 5;
    decimFactorRow = 5;
    decimFactorCol = 5;    
    %%
    [R C] = size(vel_Values);
    RV = borderOffset:decimFactorRow:(R-borderOffset);   
    CV = borderOffset:decimFactorCol:(C-borderOffset);
    [Y X] = meshgrid(CV,RV);
end

tmp = vel_Values(RV,CV);
tmp = tmp.*scaleFactor;
vel_Lines = [Y(:), X(:), Y(:)+real(tmp(:)),  X(:)+imag(tmp(:))];

== matlab function IDMF_datagenerator/Optical Flow Lines Calculation/Optical Flow Lines/Optical Flow Lines ==
  data: vel_Values input; vel_Lines output; scaleFactor parameter size=1
function vel_Lines=OpticalFlowLines(vel_Values, scaleFactor) 

% Generates the coordinate points of optical flow lines

persistent first_time;
persistent X;
persistent Y;
persistent RV;
persistent CV;
if isempty(first_time)
    first_time     = 1;
    %% user may change the following three parameters
    borderOffset   = 5;
    decimFactorRow = 5;
    decimFactorCol = 5;    
    %%
    [R C] = size(vel_Values);
    RV = borderOffset:decimFactorRow:(R-borderOffset);   
    CV = borderOffset:decimFactorCol:(C-borderOffset);
    [Y X] = meshgrid(CV,RV);
end

tmp = vel_Values(RV,CV);
tmp = tmp.*scaleFactor;
vel_Lines = [Y(:), X(:), Y(:)+real(tmp(:)), X(:)+imag(tmp(:))];

== matlab function IDMF_datagenerator/ Optical Flow Algorithm for Obstacle Avoidance/flowdiff/FlowDifferences ==
  data: flowDifference output; vleftflow output; vrightflow output; cmd output; image input
function [flowDifference,vleftflow, vrightflow,cmd] = calculatethedifference(image)

% Image Preprocessing
image = flip(image, 1);

% Image Width
width = size(image,2);

% Calculate optical flow on right-half and the left-half of the image
VLeftFlow = image(:, 1:width/2); 
VRightFlow = image(:, width/2:width);

% Sum to get the total Optical Flow on the right-half and on left-half
vleftflow = sum(VLeftFlow(:));
vrightflow = sum(VRightFlow(:));

% Find the difference of the flow between the two halves
flowDifference = (vleftflow - vrightflow);

% Steer in the direction that has less optical flow which implies less 
% obstacles
if flowDifference>0
    cmd=uint8('Steering to Left ');
else
    cmd=uint8('Steering to Right');
end

== matlab function IDMF_datagenerator/ Optical Flow Algorithm for Obstacle Avoidance/flowdiff_down/FlowDifferences2 ==
  data: flowDifference output; image input
function flowDifference = calculatethedifference(image)

% Image Preprocessing
image = flip(image, 1);

% Image Width
% width = size(image,2);
length = size(image,1);

% Calculate optical flow on right-half and the left-half of the image
VUpFlow = image(length/2:length,:); 
VDownFlow = image(1:length/2, :);

% Sum to get the total Optical Flow on the right-half and on left-half
vupflow = sum(VUpFlow(:));
vdownflow = sum(VDownFlow(:));

% Find the difference of the flow between the two halves
flowDifference = (vupflow - vdownflow);

% Steer in the direction that has less optical flow which implies less 
% obstacles

== matlab function IDMF_datagenerator/Optical Flow Lines Calculation1/MATLAB Function1 ==
  data: points input; vel_Lines output int32 size=[50 4]; vel_points output int32 size=[50 2]
function [vel_Lines, vel_points]=OpticalFlowLines(points)
%persistent vel_Lines;

orderedpointsog = sortrows(points);
X = [];
Y = [];
shiftX = [];
shiftY=[];

%|| orderedpoints(i,1)==orderedpoints(i+1,1)+1 || orderedpoints(i,1)==orderedpoints(i+1,1)-1)
for i = 1:2:length(points)-1
    if i ==1 && orderedpointsog(i,1)==orderedpointsog(i+1,1) 
        X = [X ;orderedpointsog(i,1)];
        Y = [Y ;orderedpointsog(i,2)];
        shiftX = [shiftX ;orderedpointsog(i+1,1)];
        shiftY = [shiftY ;orderedpointsog(i+1,2)];
    else
        if i ~=1 && (orderedpointsog(i,1)==orderedpointsog(i+1,1)|| orderedpointsog(i,1)==orderedpointsog(i+1,1)+1 || orderedpointsog(i,1)==orderedpointsog(i+1,1)-1 ...
                || orderedpointsog(i,1)==orderedpointsog(i+1,1)+2 || orderedpointsog(i,1)==orderedpointsog(i+1,1)-2)
        X = [X ;orderedpointsog(i,1)];
        Y = [Y ;orderedpointsog(i,2)];
        shiftX = [shiftX ;orderedpointsog(i+1,1)];
        shiftY = [shiftY ;orderedpointsog(i+1,2)];
        
        elseif i~=1 &&  (orderedpointsog(i,1)==orderedpointsog(i-1,1)|| orderedpointsog(i,1)==orderedpointsog(i-1,1)+1 || orderedpointsog(i,1)==orderedpointsog(i-1,1)-1 ...
                || orderedpointsog(i,1)==orderedpointsog(i-1,1)+2 || orderedpointsog(i,1)==orderedpointsog(i-1,1)-2)
        X = [X ;orderedpointsog(i,1)];
        Y = [Y ;orderedpointsog(i,2)];
        shiftX = [shiftX ;orderedpointsog(i-1,1)];
        shiftY = [shiftY ;orderedpointsog(i-1,2)];
    end
   end


end
vel_points = [X(:), Y(:); shiftX(:),  shiftY(:) ];
vel_Lines = [X(:), Y(:), shiftX(:),  shiftY(:)];

== matlab function IDMF_datagenerator/ Optical Flow Algorithm for Obstacle Avoidance/Optical flow algorithm and PID Controller for landing/DronePositionEstimation.DroneLandingnoZ/Landing/Subsystem/Subsystem/MATLAB Function ==
  settings: updateMethod=DISCRETE
  data: u input; y output; resetp output
function [y,resetp] = fcn(u)
persistent oldd;
persistent resetparam;
if isempty(oldd)
    oldd=u;
end
if isempty(resetparam)
    resetparam=0;
end
if u ==0
    y=oldd;
    resetparam=resetparam+1;
else
    y=u;
    if resetparam<30
    resetparam=0;
    end
end
oldd = y;
resetp=resetparam;

== matlab function IDMF_datagenerator/ Optical Flow Algorithm for Obstacle Avoidance/Subsystem/length ==
  data: lines input; l1 output size=25; oldlines input; l2 output size=25; N output
function [l1,l2,N] = fcn(lines, oldlines)
l1=single([]);
l2=single([]);
persistent x;

if isempty(x)
    x=lines;
end
oldines=x;
N = 0;
if isempty(nonzeros(oldlines))
    oldlines=lines;
end
if length(lines)<length (oldlines)
for i = 1: length(lines)
    for j = i:length(oldlines)
        if abs(lines(i,1) + lines(i,3) - oldlines(j,3) -oldlines(j,1))<=5 && N~=i
           if norm(lines(i,1:2)-lines(i,3:4))~=0 && norm(oldlines(i,1:2)-oldlines(i,3:4))~=0
            l1 = [l1 ;norm(lines(i,1:2)-lines(i,3:4))];
            l2 = [l2; norm(oldlines(j,1:2)-oldlines(j,3:4))];
            N = N+1;
           end
        end
    end
end
else
for i = 1: length(oldlines)
    for j = i:length(lines)
        if abs(oldlines(i,1) + oldlines(i,3) - lines(j,3) -lines(j,1))<=5  && N~=i
           if norm(lines(i,1:2)-lines(i,3:4))~=0 && norm(oldlines(i,1:2)-oldlines(i,3:4))~=0
            l1 = [l1 ;norm(lines(j,1:2)-lines(j,3:4))];
            l2 = [l2; norm(oldlines(i,1:2)-oldlines(i,3:4))];
            N = N+1;
           end
        end
    end
end
end
x=lines;

== matlab function IDMF_datagenerator/ Optical Flow Algorithm for Obstacle Avoidance/Optical flow algorithm and PID Controller for landing/DronePositionEstimation.DroneLandingnoZ/Landing/Subsystem/Subsystem/MATLAB Function1 ==
  data: u input; y output
function y = fcn(u)
if isnan(u)
    y=0;
else
y = u;
end
end

== matlab function IDMF_datagenerator/ Optical Flow Algorithm for Obstacle Avoidance/Optical flow algorithm and PID Controller for landing/DronePositionEstimation.DroneLandingnoZ/Landing/Subsystem/Subsystem1/MATLAB Function ==
  settings: updateMethod=DISCRETE
  data: resetp input; opz output; calcz input; currentz input; stp output; x1 output
function [opz,stp,x1] = fcn(resetp,calcz,currentz)

persistent zval;
persistent stop;
persistent x;
if isempty(zval)
    zval=calcz;
end
if isempty(stop)
    stop=0;
end
if isempty(x)
    x=0;
end
if resetp >30
    if ((zval-x)<=0.4)
            x=x-0.005;
            opz=x;
    else 
        stop =1;
        opz=x;
    end
else 
    if zval~=x && x~=0
        zval=x;
        opz=x;
    else
    zval=calcz;
    opz=zval;
    x=zval;
    end
end
stp=stop;
x1=x;

== matlab function IDMF_datagenerator/ Optical Flow Algorithm for Obstacle Avoidance/Subsystem/MATLAB Function1 ==
  settings: updateMethod=DISCRETE  sampleTime=0.01
  data: videoFrameGray input; newFeaturePointLocations output size=[50 2]; featurePointLocations input; numberOfFeaturePoints output; Reset output; oldInliers output size=[50 2]
% Function for tracking face and feature points
%
% Copyright 2016 The MathWorks, Inc.
function [newFeaturePointLocations, numberOfFeaturePoints,Reset, oldInliers]   = trackPoints(videoFrameGray, featurePointLocations)

persistent pointTracker
persistent oldPoints
% persistent bboxPoints
persistent first_time
persistent numPts
% persistent vel_lines
% persistent N
reset = 0;
x=0;
x1=single(zeros(50,2));
% Create the point tracker object.
if isempty(pointTracker)
    pointTracker = vision.PointTracker('MaxBidirectionalError', 10,'MaxIterations',50);
end
% 
% if isempty(bboxPoints)
%     bboxPoints = [0 0];
% end 

if isempty(oldPoints)
    oldPoints = single(zeros(50,2));
end      

if isempty(numPts)
    numPts = 0;
end

% if isempty(N)
%     N = 0;
% end
% 
% if isempty(vel_lines)
%     vel_lines = single(zeros(25,4));
% end

if isempty (reset)
    reset=0;
end

% Initialize tracker with dummy points
if isempty(first_time)
   initialize(pointTracker, single([10 10]),videoFrameGray);
   first_time = 0;
end

if numPts ==0 
    if featurePointLocations~=single(zeros(50,2))
        % Re-initialize the point tracker if a face has been detected and
        % feature points obtained.
        newFeaturePointLocations = featurePointLocations;
        numPts = size(newFeaturePointLocations,1);
        
        if ~pointTracker.isLocked
            initialize(pointTracker, newFeaturePointLocations,videoFrameGray);
        end
 
        %step(pointTracker, videoFrameGray);
        setPoints(pointTracker, newFeaturePointLocations);
        
        % Save a copy of the points.
        oldPoints = newFeaturePointLocations;
        oldInliers = oldPoints;
        % Convert the rectangle represented as [x, y, w, h] into an
        % M-by-2 matrix of [x,y] coordinates of the four corners. This
        % is needed to be able to transform the bounding box to display
        % the orientation of the face.
%         bboxPoints = bbox2points(bBox(1, :));
%         bBoxCornerPts = bboxPoints;
    else
%         bBoxCornerPts = [];
        newFeaturePointLocations = single(zeros(25,2));
        numPts=0;
        oldInliers = single(zeros(25,2));
    end

else
    % Tracking mode. 
    [newFeaturePointLocations, isFound] = step(pointTracker, videoFrameGray);
    assert(size(newFeaturePointLocations, 1) < 500);
    visiblePoints = newFeaturePointLocations(isFound, :);
    oldInliers = oldPoints(isFound, :);
    numPts = size(oldInliers,1);
    numPts1 = size(visiblePoints, 1);

    if numPts1>=30 && numPts>=30
        %       if numPts1>=45 abs(numPts1 -numPts) <= 5
        % Estimate the geometric transformation between the old points
        % and the new points.
%         [xform, inlierIdx] = estimateGeometricTransform2D(...
%             oldInliers, visiblePoints, 'similarity', 'MaxDistance', 20);
%         visiblePoints = visiblePoints(inlierIdx, :);

%         % Apply the transformation to the bounding box.
%         bboxPoints = double(transformPointsForward(xform, bboxPoints));
%         bBoxCornerPts = bboxPoints;

        % Assign the visible feature points
        assert(size(visiblePoints, 1) < 500);
        newFeaturePointLocations = visiblePoints;
        numPts=size(newFeaturePointLocations,1);

        % Reset the points.
        oldPoints = visiblePoints;
        setPoints(pointTracker, oldPoints);
    else
%         bBoxCornerPts = [];
%         newFeaturePointLocations = single([]);  
%         numPts=0;
        reset =1 ;
        if featurePointLocations~=single(zeros(50,2))
            % Re-initialize the point tracker if a face has been detected and
            % feature points obtained.
            % 480x320

%             x1=featurePointLocations(:,1)>100 & featurePointLocations(:,1)<380;
%             newFeaturePointLocations=featurePointLocations(x1,:);
%             
%             y1=newFeaturePointLocations(:,2)>80 & newFeaturePointLocations(:,2)<240;
%             newFeaturePointLocations=newFeaturePointLocations(y1,:);

            newFeaturePointLocations=featurePointLocations;
%             newFeaturePointLocations = padarray(featurePointLocations,50-length(featurePointLocations),0,'post');
%             numPts = size(newFeaturePointLocations,1)
            
            if ~pointTracker.isLocked
            initialize(pointTracker, newFeaturePointLocations,videoFrameGray);
            end  

            step(pointTracker, videoFrameGray);
            numPts = size(newFeaturePointLocations,1);
            setPoints(pointTracker, newFeaturePointLocations);
            
            % Save a copy of the points.
            oldPoints = newFeaturePointLocations;
            oldInliers = oldPoints;

        else

            newFeaturePointLocations = single(zeros(25,2));
            numPts=0;

        end

    end

end

numberOfFeaturePoints = numPts;
Reset=reset;

== matlab function IDMF_datagenerator/ Optical Flow Algorithm for Obstacle Avoidance/Subsystem/MATLAB Function3 ==
  data: y output size=[50 2]; u input
function y = fcn(u)
if ~isempty(u)
    points = detectFASTFeatures(u);
    points = points.selectStrongest(25);
    y=points.Location;
else
    y = single([]);
end
